simulink model "untitled"  (R2022a)
settings: Solver=VariableStepAuto  StartTime=0.0  StopTime=182  RelTol=1e-3
model workspace: external: MATLAB File C:\Users\bigba\OneDrive\Documenti\GitHub\glucose-minimal-model\code\parameters.m (data not in the file)
values from neighbouring files (symbols this model uses):
  G0 = 279    [glucose_minimal_model.m]    (also in parameters.m)
  Gb = 93    [glucose_minimal_model.m]    (also in parameters.m)
  Ib = 11    [glucose_minimal_model.m]    (also in parameters.m)
  insuline = tgi(:,3)    [glucose_minimal_model.m]    (also in parameters.m)
  k = 0.025    [glucose_minimal_model.m]    (also in parameters.m)
  Sg = 2.6E-2    (= 0.026)    [glucose_minimal_model.m]    (also in parameters.m)
  Si = 5.0e-4    (= 0.0005)    [glucose_minimal_model.m]    (also in parameters.m)
  time = tgi(:,1)    [glucose_minimal_model.m]    (also in parameters.m)
settings Model: Creator=bigba  LastModifiedBy=bigba

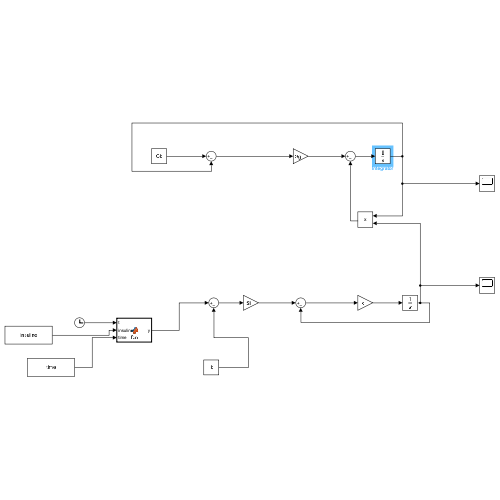
[thumbnail: Simulink's stored preview of the top-level diagram]
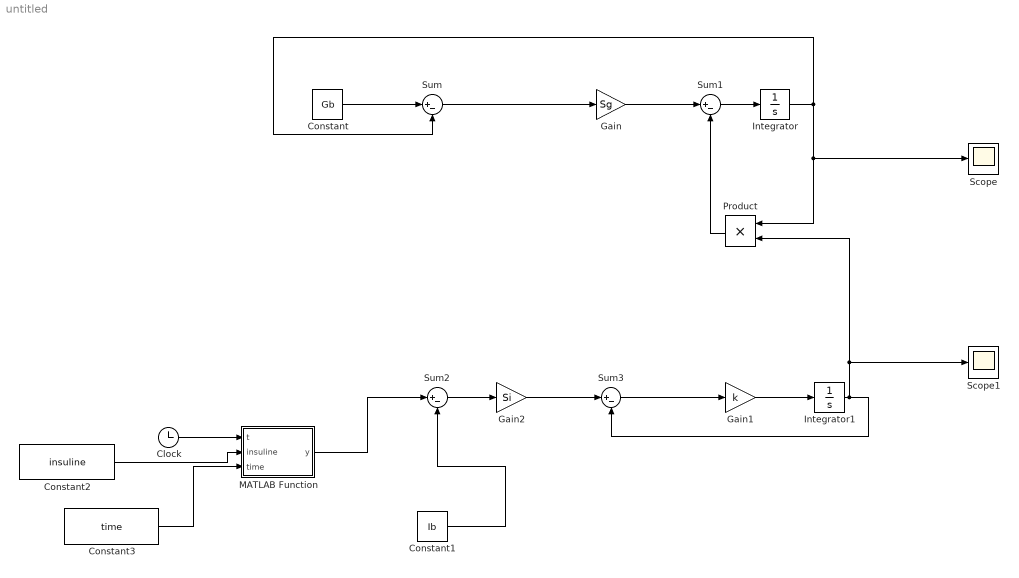
== system untitled ==
  Clock : Clock
  Constant : Constant  Value=Gb
  Constant1 : Constant  Value=Ib
  Constant2 : Constant  Value=insuline
  Constant3 : Constant  Value=time
  Gain : Gain  Gain=Sg
  Gain1 : Gain  Gain=k
  Gain2 : Gain  Gain=Si
  Integrator : Integrator  InitialCondition=G0
  Integrator1 : Integrator
  MATLAB Function : MATLAB Function  TreatAsAtomicUnit=on
  Product : Product
  Scope : Scope
  Scope1 : Scope
  Sum{,1..3} (4 alike) : Sum  Inputs=|+-
  wires:
  Constant/1 -> Sum/1
  Sum/1 -> Gain/1
  Gain/1 -> Sum1/1
  Sum1/1 -> Integrator/1
  Integrator/1 -> Scope/1, Product/1, Sum/2
  Product/1 -> Sum1/2
  Constant1/1 -> Sum2/2
  MATLAB Function/1(y) -> Sum2/1
  Sum2/1 -> Gain2/1
  Gain2/1 -> Sum3/1
  Sum3/1 -> Gain1/1
  Gain1/1 -> Integrator1/1
  Integrator1/1 -> Scope1/1, Product/2, Sum3/2
  Clock/1 -> MATLAB Function/1(t)
  Constant2/1 -> MATLAB Function/2(insuline)
  Constant3/1 -> MATLAB Function/3(time)

== matlab function untitled/MATLAB Function ==
  data: t input; y output; insuline input; time input
function y = fcn(t,insuline,time)
y=interp1(time,insuline,t);
